simulink library "cooling_lib"  (R2022b)
settings: Solver=VariableStepAuto  StartTime=0.0  StopTime=10.0  RelTol=1e-3
undefined symbols (not defined in the file): raptor_get_param_eval, raptor_xcp_function
libraries: Raptor_lib x18, simulink x6
settings Model: Creator=serga  LastModifiedBy=serga

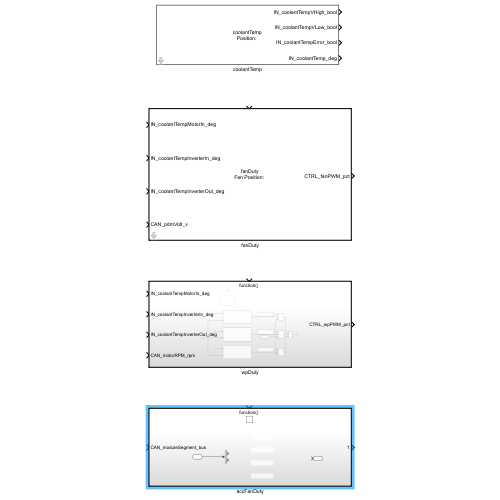
[thumbnail: Simulink's stored preview of the top-level diagram]
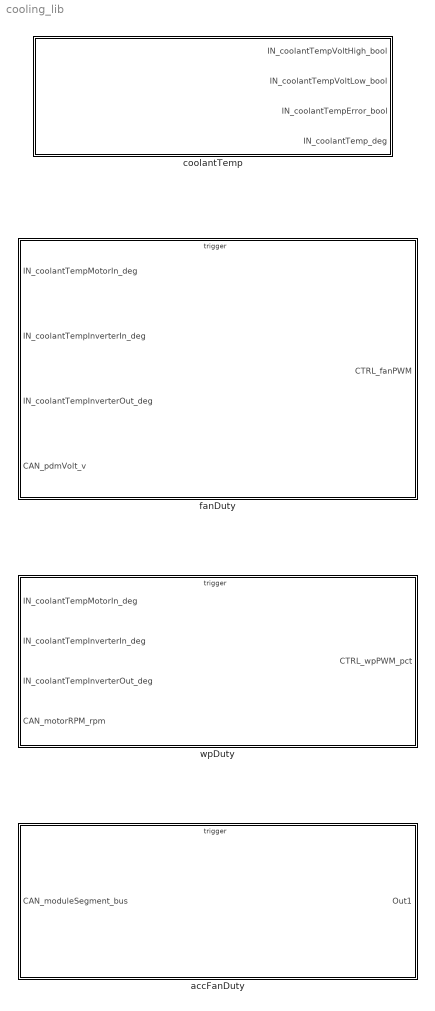
== system cooling_lib ==
  accFanDuty : Subsystem
  coolantTemp : Subsystem  mask{pos=''}
      mask prompts: pos "Position"
      mask Display:
      | disp(['coolantTemp\n'...
      |     'Position: ' pos]);
      | port_label('output', 1, ['IN_coolantTempVHigh' pos '_bool']);
      | port_label('output', 2, ['IN_coolantTempVLow' pos '_bool']);
      | port_label('output', 3, ['IN_coolantTempError' pos '_bool']);
      | port_label('output', 4, ['IN_coolantTemp' pos '_deg']);
  fanDuty : Subsystem  mask{pos=''}
      mask prompts: pos "Position"
      mask Display:
      | disp(['fanDuty\n'...
      |     'Fan Position: ' pos]);
      | port_label('input', 1, 'IN_coolantTempMotorIn_deg');
      | port_label('input', 2, 'IN_coolantTempInverterIn_deg');
      | port_label('input', 3, 'IN_coolantTempInverterOut_deg');
      | port_label('input', 4, 'CAN_pdmVolt_v');
      | port_label('output', 1, ['CTRL_fan' pos 'PWM_pct']);
  wpDuty : Subsystem

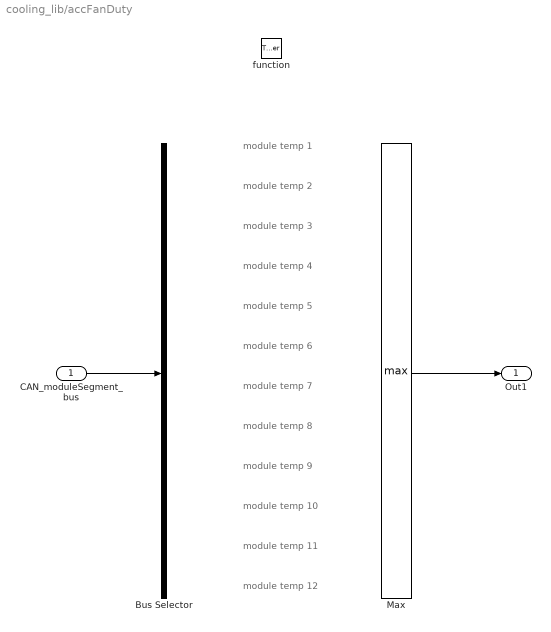
== system cooling_lib/accFanDuty ==
  note: module temp 1
  note: module temp 2
  note: module temp 3
  note: module temp 4
  note: module temp 5
  note: module temp 6
  note: module temp 7
  note: module temp 8
  note: module temp 9
  note: module temp 10
  note: module temp 11
  note: module temp 12
  CAN_moduleSegment_bus : Inport
  function : TriggerPort  TriggerType=function-call  VariantControl=(inherit)
  Bus Selector : BusSelector  OutputSignals=signal1,signal2
  Max : MinMax  Function=max  Inputs=12
  Out1 : Outport
  wires:
  CAN_moduleSegment_bus/1 -> Bus Selector/1
  Max/1 -> Out1/1

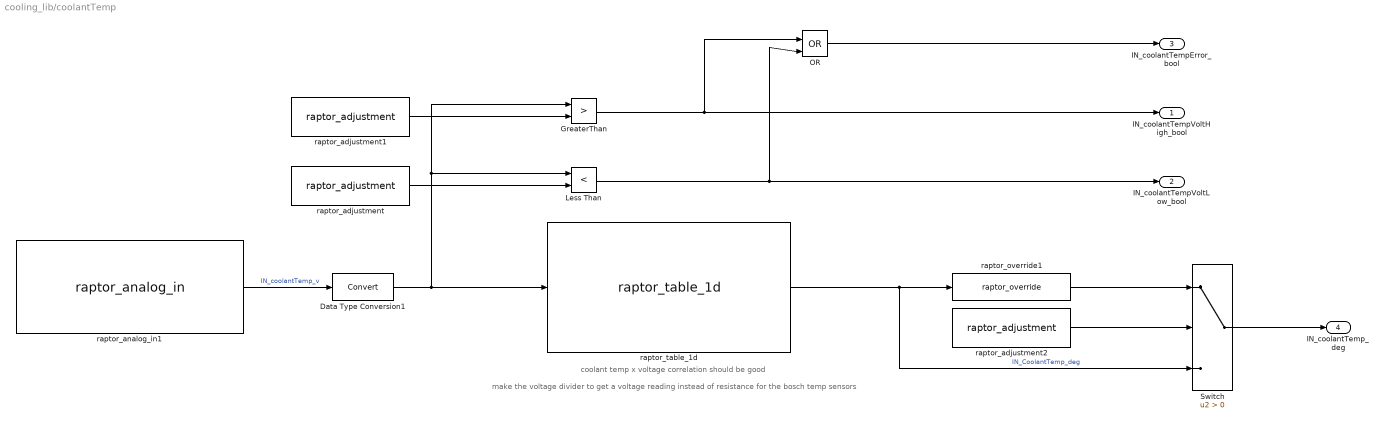
== system cooling_lib/coolantTemp ==
  note: coolant temp x voltage correlation should be good
  note: make the voltage divider to get a voltage reading instead of resistance for the bosch temp sensors
  Data Type Conversion1 : DataTypeConversion  SaturateOnIntegerOverflow=off  RndMeth=Floor
  GreaterThan : RelationalOperator  Operator=>  OutDataTypeStr=boolean  RndMeth=Simplest  InputSameDT=off
  Less Than : RelationalOperator  Operator=<  OutDataTypeStr=boolean  RndMeth=Simplest  InputSameDT=off
  OR : Logic  Operator=OR  IconShape=distinctive  AllPortsSameDT=off  OutDataTypeStr=boolean
  Switch : Switch  Criteria=u2 > Threshold  SaturateOnIntegerOverflow=off  InputSameDT=off
  raptor_adjustment : Raptor_lib/Data Storage/raptor_adjustment  paramName=['IN_coolantTempLow' pos '_v']  nameSource=Parameter  initValue=0.5  dataType=single  storage=Calibration  calDispType=Number  calEnum={'False', 'True'}  calGain=1.0  calOffset=0.0  calMax=inf  calMin=-inf  calFormat='-1'  calUnit=''  calHelp=''  calAccess=1  calFunction=raptor_xcp_function(gcb)  calDispHeaders=off  calColHeaders={'Col1' 'Col2' 'Col3'}  calRowHeaders={'Row1' 'Row2' 'Row3'}
      settings: SourceProductName=Raptor
  raptor_adjustment1 : Raptor_lib/Data Storage/raptor_adjustment  paramName=['IN_coolantTempHigh' pos '_v']  nameSource=Parameter  initValue=4.5  dataType=single  storage=Calibration  calDispType=Number  calEnum={'False', 'True'}  calGain=1.0  calOffset=0.0  calMax=inf  calMin=-inf  calFormat='-1'  calUnit=''  calHelp=''  calAccess=1  calFunction=raptor_xcp_function(gcb)  calDispHeaders=off  calColHeaders={'Col1' 'Col2' 'Col3'}  calRowHeaders={'Row1' 'Row2' 'Row3'}
      settings: SourceProductName=Raptor
  raptor_adjustment2 : Raptor_lib/Data Storage/raptor_adjustment  paramName=['IN_coolantTemp' pos '_bool']  nameSource=Parameter  initValue=0.00  dataType=boolean  storage=Calibration  calDispType=Number  calEnum={'False', 'True'}  calGain=1.0  calOffset=0.0  calMax=inf  calMin=-inf  calFormat='-1'  calUnit=''  calHelp=''  calAccess=1  calFunction=raptor_xcp_function(gcb)  calDispHeaders=off  calColHeaders={'Col1' 'Col2' 'Col3'}  calRowHeaders={'Row1' 'Row2' 'Row3'}
      settings: SourceProductName=Raptor
  raptor_analog_in1 : Raptor_lib/Input & Output/raptor_analog_in  resourceValues=INPUT2|INPUT3|INPUT4|INPUT5|INPUT6|INPUT7|INPUT8|INPUT9|INPUT10|INPUT11|INPUT12|INPUT13|INPUT14|INPUT15|INPUT16|INPUT17|INPUT18|INPUT19|INPUT20|INPUT21|INPUT22|INPUT23|INPUT24|INPUT25|INPUT26|INPUT27|INPUT28|INPUT29|INPUT30|INPUT31|INPUT32|(None)  resource=INPUT2  pullUDValues=2.15k PU  pullUD=2.15k PU  rangeValues=0 - 5 V  range=0 - 5 V  filterrateValues=[]  filterrate='RAPTOR MASK DEFAULT'  resolutionValues=[]  resolution=[]
      settings: SourceProductName=Raptor
  raptor_override1 : Raptor_lib/Data Storage/raptor_override  paramName=['IN_coolantTemp' pos '_deg']  nameSource=Parameter  measurement=Output  calDispType=Number  calEnum={'False', 'True'}  calGain=1.0  calOffset=0.0  calMax=inf  calMin=-inf  calFormat='-1'  calUnit=''  calHelp=''  calAccess=1  calFunction="[raptor_xcp_function(gcb) '|'  'Override']"
      settings: SourceProductName=Raptor
  raptor_table_1d : Raptor_lib/Table Lookup/raptor_table_1d  dataName=['IN_coolantTempVToDeg' pos]  initValue=[150 140 130 120 110 100 90 80 70 60 50 40 30 20 10 0 -10 -20 -30 -40]  dataType=double  storage=Calibration  initValueX=[0.2267 0.2793 0.3452 0.4303 0.5357 0.6741 0.8420 1.0604 1.3325 1.6592 2.0501 2.4737 2.9360 3.3784 3.7981 4.1545 4.4338 4.6399 4.7803 4.8710]  dataTypeXY=double  storageXY=Calibration  calVisible=on  showTable=on  calGain=1.0  calOffset=0.0  calMax=Inf  calMin=-Inf  calFormat='-1'  calUnit='Deg_C'  calHelp=''  showBreakpoint=on  dataNameX=[]  calGainX=1.0  calOffsetX=0.0  calMaxX=Inf  calMinX=-Inf  calFormatX='-1'  calUnitX='V'  calHelpX=''  calAccess=1  calFunction=raptor_xcp_function(gcb)  measureEnable=off  mName=['Data1D_Output']
      settings: SourceProductName=Raptor
  IN_coolantTempVoltHigh_bool : Outport  OutDataTypeStr=boolean
  IN_coolantTempVoltLow_bool : Outport  Port=2  OutDataTypeStr=boolean
  IN_coolantTempError_bool : Outport  Port=3  OutDataTypeStr=boolean
  IN_coolantTemp_deg : Outport  Port=4  OutDataTypeStr=double
  wires:
  raptor_override1/1 -> Switch/1
  OR/1 -> IN_coolantTempError_bool/1
  raptor_adjustment2/1 -> Switch/2
  raptor_analog_in1/1 -> Data Type Conversion1/1  "IN_coolantTemp_v"
  raptor_adjustment/1 -> Less Than/2
  raptor_table_1d/1 -> raptor_override1/1, Switch/3  "IN_CoolantTemp_deg"
  raptor_adjustment1/1 -> GreaterThan/2
  Switch/1 -> IN_coolantTemp_deg/1
  Less Than/1 -> IN_coolantTempVoltLow_bool/1, OR/2
  GreaterThan/1 -> OR/1, IN_coolantTempVoltHigh_bool/1
  Data Type Conversion1/1 -> GreaterThan/1, Less Than/1, raptor_table_1d/1

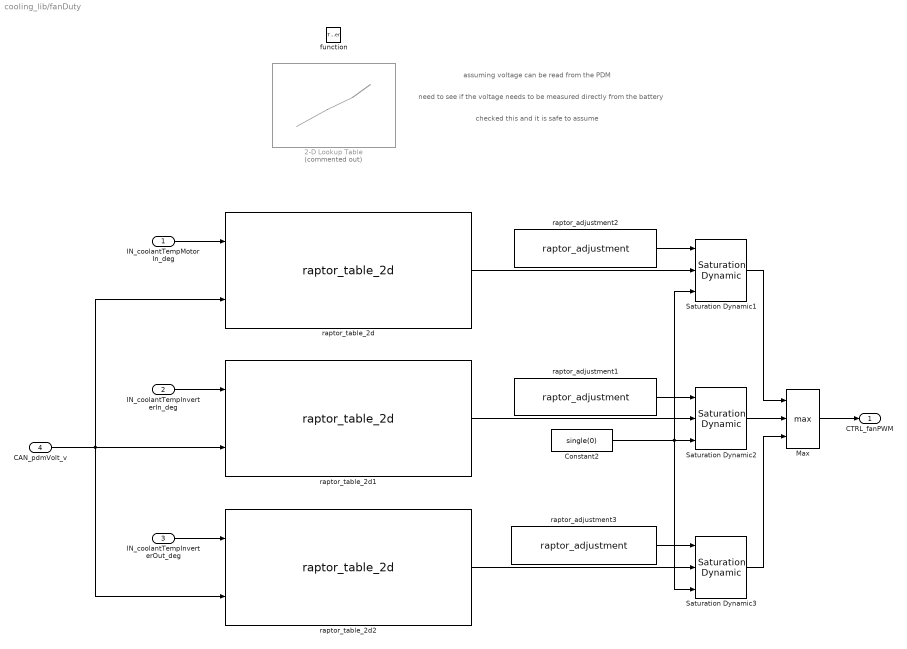
== system cooling_lib/fanDuty ==
  note: checked this and it is safe to assume
  note: need to see if the voltage needs to be measured directly from the battery
  note: assuming voltage can be read from the PDM
  IN_coolantTempMotorIn_deg : Inport
  IN_coolantTempInverterIn_deg : Inport  Port=2
  IN_coolantTempInverterOut_deg : Inport  Port=3
  CAN_pdmVolt_v : Inport  Port=4
  function : TriggerPort  TriggerType=function-call  VariantControl=(inherit)
  2-D Lookup Table : Lookup_n-D  Commented=on  LookupTableObject=''  BreakpointsForDimension1=[0;60;75;75.1;82;82.1;85;85.1;100;100.1;150]  BreakpointsForDimension2=[0 8 9 10 10.5 11 11.9 12 13 13.7 13.8 13.9 14.2 14.5]  BreakpointsForDimension1FirstPoint=10  BreakpointsForDimension2FirstPoint=10  BreakpointsForDimension1Spacing=12  BreakpointsForDimension2Spacing=12  IndexSearchMethod=Evenly spaced points  Table=[0 0 0 0 0 0 0 0 0 0 0 0 0 0;0 0 0 0 0 0 0 0 0 0 0 0 0 0;0 0 0 0 0 0 0 0 0 0 0 0 0 25;0 15 15 15 15 15 15 15 15 15 30 30 30 30;0 15 15 15 15 15 15 15 15 15 50 50 50 50;0 15 15 15 25 25 25 25 25 25 65 65 65 65;0 75 75 75 75 75 75 75 75 75 75 75 75 75;0 100 100 100 100 100 100 100 100 100 100 100 100 100;0 100 100 100 100 100 100 100 100 100 100 100 100 100;0 100 100 100 100 100 100 100 100 100 100 100 100 100;0 100 100 100 100 100 100 100 100 100 100 100 100 100]  InterpMethod=Flat  DiagnosticForOutOfRangeInput=Error  InternalRulePriority=Speed  RndMeth=Simplest
      settings: InputPortMap=u0,u1
  Constant2 : Constant  Value=single(0)
  Max : MinMax  Function=max  Inputs=3
  Saturation Dynamic1 : simulink/Discontinuities/Saturation Dynamic  OutMin=[]  OutMax=[]  OutDataTypeStr=Inherit: Same as second input  OutDataType=fixdt(1, 16)  OutScaling=2^-10  DoSatur=off
  Saturation Dynamic2 : simulink/Discontinuities/Saturation Dynamic  OutMin=[]  OutMax=[]  OutDataTypeStr=Inherit: Same as second input  OutDataType=fixdt(1, 16)  OutScaling=2^-10  DoSatur=off
  Saturation Dynamic3 : simulink/Discontinuities/Saturation Dynamic  OutMin=[]  OutMax=[]  OutDataTypeStr=Inherit: Same as second input  OutDataType=fixdt(1, 16)  OutScaling=2^-10  DoSatur=off
  raptor_adjustment1 : Raptor_lib/Data Storage/raptor_adjustment  paramName=['CTRL_upperThreshCoolantInverterIn' pos]  nameSource=Parameter  initValue=100  dataType=single  storage=Calibration  calDispType=Number  calEnum={'False', 'True'}  calGain=1.0  calOffset=0.0  calMax=inf  calMin=-inf  calFormat='-1'  calUnit=''  calHelp=''  calAccess=1  calFunction=raptor_xcp_function(gcb)  calDispHeaders=off  calColHeaders={'Col1' 'Col2' 'Col3'}  calRowHeaders={'Row1' 'Row2' 'Row3'}
      settings: SourceProductName=Raptor
  raptor_adjustment2 : Raptor_lib/Data Storage/raptor_adjustment  paramName=['CTRL_upperThreshCoolantMotorIn' pos]  nameSource=Parameter  initValue=100  dataType=single  storage=Calibration  calDispType=Number  calEnum={'False', 'True'}  calGain=1.0  calOffset=0.0  calMax=inf  calMin=-inf  calFormat='-1'  calUnit=''  calHelp=''  calAccess=1  calFunction=raptor_xcp_function(gcb)  calDispHeaders=off  calColHeaders={'Col1' 'Col2' 'Col3'}  calRowHeaders={'Row1' 'Row2' 'Row3'}
      settings: SourceProductName=Raptor
  raptor_adjustment3 : Raptor_lib/Data Storage/raptor_adjustment  paramName=['CTRL_upperThreshCoolantInverterOut' pos]  nameSource=Parameter  initValue=100  dataType=single  storage=Calibration  calDispType=Number  calEnum={'False', 'True'}  calGain=1.0  calOffset=0.0  calMax=inf  calMin=-inf  calFormat='-1'  calUnit=''  calHelp=''  calAccess=1  calFunction=raptor_xcp_function(gcb)  calDispHeaders=off  calColHeaders={'Col1' 'Col2' 'Col3'}  calRowHeaders={'Row1' 'Row2' 'Row3'}
      settings: SourceProductName=Raptor
  raptor_table_2d : Raptor_lib/Table Lookup/raptor_table_2d  dataName=['CTRL_coolantTempMotorInTo' pos 'Duty']  initValue=[0 0 0 0 0 0 0 0 0 0 0 0 0 0;0 0 0 0 0 0 0 0 0 0 0 0 0 0;0 0 0 0 0 0 0 0 0 0 0 0 0 25;0 15 15 15 15 15 15 15 15 15 30 30 30 30;0 15 15 15 15 15 15 15 15 15 50 50 50 50;0 15 15 15 25 25 25 25 25 25 65 65 65 65;0 75 75 75 75 75 75 75 75 75 75 75 75 75;0 100 100 100 100 100 100 100 100 100 100 100 100 100;0 100 100 100 100 100 100 100 100 100 100 100 100 100;0 100 100 100 100 100 100 100 100 100 100 100 100 100;0 100 100 100 100 100 100 100 100 100 100 100 100 100]  dataType=double  storage=Calibration  initValueX=[0 8 9 10 10.5 11 11.9 12 13 13.7 13.8 13.9 14.2 14.5]  initValueY=[0;60;75;75.1;82;82.1;85;85.1;100;100.1;150]  dataTypeXY=double  storageXY=Calibration  calVisible=on  showTable=off  calGain=1.0  calOffset=0.0  calMax=Inf  calMin=-Inf  calFormat='-1'  calUnit=''  calHelp=''  showBreakpointX=on  dataNameX=[]  calGainX=1.0  calOffsetX=0.0  calMaxX=Inf  calMinX=-Inf  calFormatX='-1'  calUnitX='pdmVolt'  calHelpX=''  showBreakpointY=on  dataNameY=[]  calGainY=1.0  calOffsetY=0.0  calMaxY=Inf  calMinY=-Inf  calFormatY='-1'  calUnitY='degC'  calHelpY=''  calAccess=1  calFunction=raptor_xcp_function(gcb)  measureEnable=off  mName=[raptor_get_param_eval(gcb,'dataName'), '_Output']
      settings: SourceProductName=Raptor
  raptor_table_2d1 : Raptor_lib/Table Lookup/raptor_table_2d  dataName=['CTRL_coolantTempInverterInTo' pos 'Duty']  initValue=[0 0 0 0 0 0 0 0 0 0 0 0 0 0;0 0 0 0 0 0 0 0 0 0 0 0 0 0;0 0 0 0 0 0 0 0 0 0 0 0 0 25;0 15 15 15 15 15 15 15 15 15 30 30 30 30;0 15 15 15 15 15 15 15 15 15 50 50 50 50;0 15 15 15 25 25 25 25 25 25 65 65 65 65;0 75 75 75 75 75 75 75 75 75 75 75 75 75;0 100 100 100 100 100 100 100 100 100 100 100 100 100;0 100 100 100 100 100 100 100 100 100 100 100 100 100;0 100 100 100 100 100 100 100 100 100 100 100 100 100;0 100 100 100 100 100 100 100 100 100 100 100 100 100]  dataType=double  storage=Calibration  initValueX=[0 8 9 10 10.5 11 11.9 12 13 13.7 13.8 13.9 14.2 14.5]  initValueY=[0;60;75;75.1;82;82.1;85;85.1;100;100.1;150]  dataTypeXY=double  storageXY=Calibration  calVisible=on  showTable=off  calGain=1.0  calOffset=0.0  calMax=Inf  calMin=-Inf  calFormat='-1'  calUnit=''  calHelp=''  showBreakpointX=on  dataNameX=[]  calGainX=1.0  calOffsetX=0.0  calMaxX=Inf  calMinX=-Inf  calFormatX='-1'  calUnitX='pdmVolt'  calHelpX=''  showBreakpointY=on  dataNameY=[]  calGainY=1.0  calOffsetY=0.0  calMaxY=Inf  calMinY=-Inf  calFormatY='-1'  calUnitY='degC'  calHelpY=''  calAccess=1  calFunction=raptor_xcp_function(gcb)  measureEnable=off  mName=[raptor_get_param_eval(gcb,'dataName'), '_Output']
      settings: SourceProductName=Raptor
  raptor_table_2d2 : Raptor_lib/Table Lookup/raptor_table_2d  dataName=['CTRL_coolantTempInverterOutTo' pos 'Duty']  initValue=[0 0 0 0 0 0 0 0 0 0 0 0 0 0;0 0 0 0 0 0 0 0 0 0 0 0 0 0;0 0 0 0 0 0 0 0 0 0 0 0 0 25;0 15 15 15 15 15 15 15 15 15 30 30 30 30;0 15 15 15 15 15 15 15 15 15 50 50 50 50;0 15 15 15 25 25 25 25 25 25 65 65 65 65;0 75 75 75 75 75 75 75 75 75 75 75 75 75;0 100 100 100 100 100 100 100 100 100 100 100 100 100;0 100 100 100 100 100 100 100 100 100 100 100 100 100;0 100 100 100 100 100 100 100 100 100 100 100 100 100;0 100 100 100 100 100 100 100 100 100 100 100 100 100]  dataType=double  storage=Calibration  initValueX=[0 8 9 10 10.5 11 11.9 12 13 13.7 13.8 13.9 14.2 14.5]  initValueY=[0;60;75;75.1;82;82.1;85;85.1;100;100.1;150]  dataTypeXY=double  storageXY=Calibration  calVisible=on  showTable=off  calGain=1.0  calOffset=0.0  calMax=Inf  calMin=-Inf  calFormat='-1'  calUnit=''  calHelp=''  showBreakpointX=on  dataNameX=[]  calGainX=1.0  calOffsetX=0.0  calMaxX=Inf  calMinX=-Inf  calFormatX='-1'  calUnitX='pdmVolt'  calHelpX=''  showBreakpointY=on  dataNameY=[]  calGainY=1.0  calOffsetY=0.0  calMaxY=Inf  calMinY=-Inf  calFormatY='-1'  calUnitY='degC'  calHelpY=''  calAccess=1  calFunction=raptor_xcp_function(gcb)  measureEnable=off  mName=[raptor_get_param_eval(gcb,'dataName'), '_Output']
      settings: SourceProductName=Raptor
  CTRL_fanPWM : Outport
  wires:
  IN_coolantTempMotorIn_deg/1 -> raptor_table_2d/1
  IN_coolantTempInverterIn_deg/1 -> raptor_table_2d1/1
  IN_coolantTempInverterOut_deg/1 -> raptor_table_2d2/1
  CAN_pdmVolt_v/1 -> raptor_table_2d/2, raptor_table_2d1/2, raptor_table_2d2/2
  Max/1 -> CTRL_fanPWM/1
  raptor_table_2d/1 -> Saturation Dynamic1/2
  Saturation Dynamic1/1 -> Max/1
  Saturation Dynamic2/1 -> Max/2
  raptor_table_2d1/1 -> Saturation Dynamic2/2
  raptor_table_2d2/1 -> Saturation Dynamic3/2
  Saturation Dynamic3/1 -> Max/3
  Constant2/1 -> Saturation Dynamic1/3, Saturation Dynamic3/3, Saturation Dynamic2/3
  raptor_adjustment2/1 -> Saturation Dynamic1/1
  raptor_adjustment1/1 -> Saturation Dynamic2/1
  raptor_adjustment3/1 -> Saturation Dynamic3/1

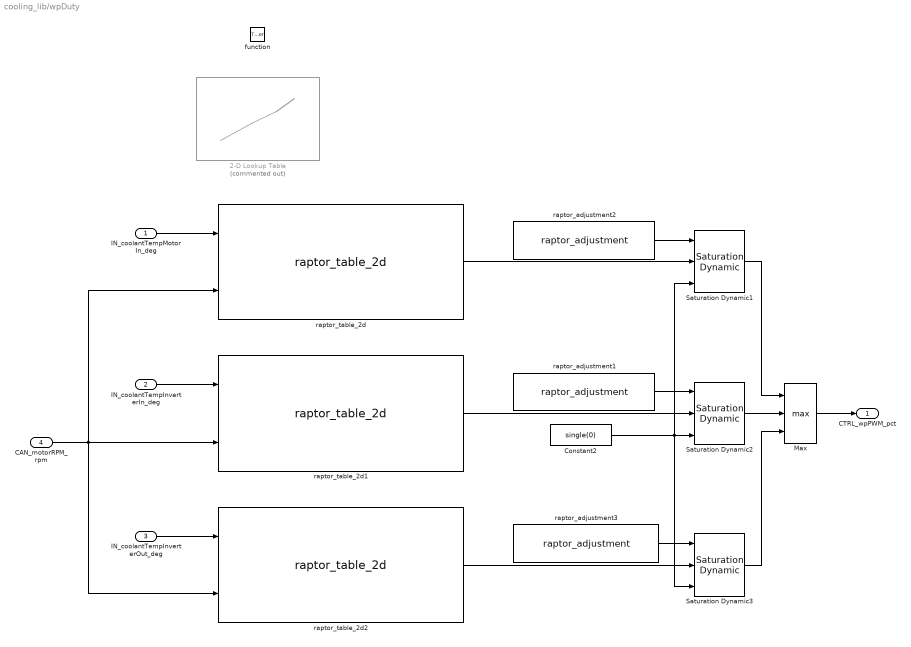
== system cooling_lib/wpDuty ==
  IN_coolantTempMotorIn_deg : Inport
  IN_coolantTempInverterIn_deg : Inport  Port=2
  IN_coolantTempInverterOut_deg : Inport  Port=3
  CAN_motorRPM_rpm : Inport  Port=4
  function : TriggerPort  TriggerType=function-call  VariantControl=(inherit)
  2-D Lookup Table : Lookup_n-D  Commented=on  LookupTableObject=''  BreakpointsForDimension1=[10;20;40;50;60;69.9;70;84.5;84.6;100;150]  BreakpointsForDimension2=[0;0;10;20;500;510;5000;15000]  BreakpointsForDimension1FirstPoint=10  BreakpointsForDimension2FirstPoint=10  BreakpointsForDimension1Spacing=12  BreakpointsForDimension2Spacing=12  IndexSearchMethod=Evenly spaced points  Table=[0 0 0 0 0 20 20 0;0 0 0 0 0 20 20 0;0 0 0 0 0 35 35 15;0 0 0 0 0 35 35 15;0 0 0 0 0 35 35 25;0 0 0 0 0 35 35 75;0 0 0 0 0 40 40 40;0 0 0 0 0 50 50 50;0 0 25 0 0 60 60 60;0 0 100 0 0 100 100 100;0 0 100 0 0 100 100 100]  InterpMethod=Flat  DiagnosticForOutOfRangeInput=Error  InternalRulePriority=Speed  RndMeth=Simplest
      settings: InputPortMap=u0,u1
  Constant2 : Constant  Value=single(0)
  Max : MinMax  Function=max  Inputs=3
  Saturation Dynamic1 : simulink/Discontinuities/Saturation Dynamic  OutMin=[]  OutMax=[]  OutDataTypeStr=Inherit: Same as second input  OutDataType=fixdt(1, 16)  OutScaling=2^-10  DoSatur=off
  Saturation Dynamic2 : simulink/Discontinuities/Saturation Dynamic  OutMin=[]  OutMax=[]  OutDataTypeStr=Inherit: Same as second input  OutDataType=fixdt(1, 16)  OutScaling=2^-10  DoSatur=off
  Saturation Dynamic3 : simulink/Discontinuities/Saturation Dynamic  OutMin=[]  OutMax=[]  OutDataTypeStr=Inherit: Same as second input  OutDataType=fixdt(1, 16)  OutScaling=2^-10  DoSatur=off
  raptor_adjustment1 : Raptor_lib/Data Storage/raptor_adjustment  paramName='CTRL_upperThreshCoolantInverterIn'  nameSource=Parameter  initValue=100  dataType=single  storage=Calibration  calDispType=Number  calEnum={'False', 'True'}  calGain=1.0  calOffset=0.0  calMax=inf  calMin=-inf  calFormat='-1'  calUnit=''  calHelp=''  calAccess=1  calFunction=raptor_xcp_function(gcb)  calDispHeaders=off  calColHeaders={'Col1' 'Col2' 'Col3'}  calRowHeaders={'Row1' 'Row2' 'Row3'}
      settings: SourceProductName=Raptor
  raptor_adjustment2 : Raptor_lib/Data Storage/raptor_adjustment  paramName='CTRL_upperThreshCoolantMotorIn'  nameSource=Parameter  initValue=100  dataType=single  storage=Calibration  calDispType=Number  calEnum={'False', 'True'}  calGain=1.0  calOffset=0.0  calMax=inf  calMin=-inf  calFormat='-1'  calUnit=''  calHelp=''  calAccess=1  calFunction=raptor_xcp_function(gcb)  calDispHeaders=off  calColHeaders={'Col1' 'Col2' 'Col3'}  calRowHeaders={'Row1' 'Row2' 'Row3'}
      settings: SourceProductName=Raptor
  raptor_adjustment3 : Raptor_lib/Data Storage/raptor_adjustment  paramName='CTRL_upperThreshCoolantInverterOut'  nameSource=Parameter  initValue=100  dataType=single  storage=Calibration  calDispType=Number  calEnum={'False', 'True'}  calGain=1.0  calOffset=0.0  calMax=inf  calMin=-inf  calFormat='-1'  calUnit=''  calHelp=''  calAccess=1  calFunction=raptor_xcp_function(gcb)  calDispHeaders=off  calColHeaders={'Col1' 'Col2' 'Col3'}  calRowHeaders={'Row1' 'Row2' 'Row3'}
      settings: SourceProductName=Raptor
  raptor_table_2d : Raptor_lib/Table Lookup/raptor_table_2d  dataName='CTRL_coolantTempMotorInToWpDuty'  initValue=[0 0 0 0 0 20 20 0;0 0 0 0 0 20 20 0;0 0 0 0 0 35 35 15;0 0 0 0 0 35 35 15;0 0 0 0 0 35 35 25;0 0 0 0 0 35 35 75;0 0 0 0 0 40 40 40;0 0 0 0 0 50 50 50;0 0 25 0 0 60 60 60;0 0 100 0 0 100 100 100;0 0 100 0 0 100 100 100]  dataType=double  storage=Calibration  initValueX=[0;0;10;20;500;510;5000;15000]  initValueY=[10;20;40;50;60;69.9;70;84.5;84.6;100;150]  dataTypeXY=double  storageXY=Calibration  calVisible=on  showTable=off  calGain=1.0  calOffset=0.0  calMax=Inf  calMin=-Inf  calFormat='-1'  calUnit=''  calHelp=''  showBreakpointX=on  dataNameX=[]  calGainX=1.0  calOffsetX=0.0  calMaxX=Inf  calMinX=-Inf  calFormatX='-1'  calUnitX='motorRPM'  calHelpX=''  showBreakpointY=on  dataNameY=[]  calGainY=1.0  calOffsetY=0.0  calMaxY=Inf  calMinY=-Inf  calFormatY='-1'  calUnitY='degC'  calHelpY=''  calAccess=1  calFunction=raptor_xcp_function(gcb)  measureEnable=off  mName=[raptor_get_param_eval(gcb,'dataName'), '_Output']
      settings: SourceProductName=Raptor
  raptor_table_2d1 : Raptor_lib/Table Lookup/raptor_table_2d  dataName='CTRL_coolantTempInverterInToWpDuty'  initValue=[0 0 0 0 0 20 20 0;0 0 0 0 0 20 20 0;0 0 0 0 0 35 35 15;0 0 0 0 0 35 35 15;0 0 0 0 0 35 35 25;0 0 0 0 0 35 35 75;0 0 0 0 0 40 40 40;0 0 0 0 0 50 50 50;0 0 25 0 0 60 60 60;0 0 100 0 0 100 100 100;0 0 100 0 0 100 100 100]  dataType=double  storage=Calibration  initValueX=[0;0;10;20;500;510;5000;15000]  initValueY=[10;20;40;50;60;69.9;70;84.5;84.6;100;150]  dataTypeXY=double  storageXY=Calibration  calVisible=on  showTable=off  calGain=1.0  calOffset=0.0  calMax=Inf  calMin=-Inf  calFormat='-1'  calUnit=''  calHelp=''  showBreakpointX=on  dataNameX=[]  calGainX=1.0  calOffsetX=0.0  calMaxX=Inf  calMinX=-Inf  calFormatX='-1'  calUnitX='motorRPM'  calHelpX=''  showBreakpointY=on  dataNameY=[]  calGainY=1.0  calOffsetY=0.0  calMaxY=Inf  calMinY=-Inf  calFormatY='-1'  calUnitY='degC'  calHelpY=''  calAccess=1  calFunction=raptor_xcp_function(gcb)  measureEnable=off  mName=[raptor_get_param_eval(gcb,'dataName'), '_Output']
      settings: SourceProductName=Raptor
  raptor_table_2d2 : Raptor_lib/Table Lookup/raptor_table_2d  dataName='CTRL_coolantTempInverterOutToWpDuty'  initValue=[0 0 0 0 0 20 20 0;0 0 0 0 0 20 20 0;0 0 0 0 0 35 35 15;0 0 0 0 0 35 35 15;0 0 0 0 0 35 35 25;0 0 0 0 0 35 35 75;0 0 0 0 0 40 40 40;0 0 0 0 0 50 50 50;0 0 25 0 0 60 60 60;0 0 100 0 0 100 100 100;0 0 100 0 0 100 100 100]  dataType=double  storage=Calibration  initValueX=[0;0;10;20;500;510;5000;15000]  initValueY=[10;20;40;50;60;69.9;70;84.5;84.6;100;150]  dataTypeXY=double  storageXY=Calibration  calVisible=on  showTable=off  calGain=1.0  calOffset=0.0  calMax=Inf  calMin=-Inf  calFormat='-1'  calUnit=''  calHelp=''  showBreakpointX=on  dataNameX=[]  calGainX=1.0  calOffsetX=0.0  calMaxX=Inf  calMinX=-Inf  calFormatX='-1'  calUnitX='motorRPM'  calHelpX=''  showBreakpointY=on  dataNameY=[]  calGainY=1.0  calOffsetY=0.0  calMaxY=Inf  calMinY=-Inf  calFormatY='-1'  calUnitY='degC'  calHelpY=''  calAccess=1  calFunction=raptor_xcp_function(gcb)  measureEnable=off  mName=[raptor_get_param_eval(gcb,'dataName'), '_Output']
      settings: SourceProductName=Raptor
  CTRL_wpPWM_pct : Outport
  wires:
  IN_coolantTempMotorIn_deg/1 -> raptor_table_2d/1
  IN_coolantTempInverterIn_deg/1 -> raptor_table_2d1/1
  IN_coolantTempInverterOut_deg/1 -> raptor_table_2d2/1
  CAN_motorRPM_rpm/1 -> raptor_table_2d2/2, raptor_table_2d1/2, raptor_table_2d/2
  raptor_adjustment1/1 -> Saturation Dynamic2/1
  Saturation Dynamic2/1 -> Max/2
  Saturation Dynamic1/1 -> Max/1
  Max/1 -> CTRL_wpPWM_pct/1
  raptor_table_2d1/1 -> Saturation Dynamic2/2
  raptor_adjustment2/1 -> Saturation Dynamic1/1
  raptor_table_2d2/1 -> Saturation Dynamic3/2
  Constant2/1 -> Saturation Dynamic2/3, Saturation Dynamic1/3, Saturation Dynamic3/3
  raptor_table_2d/1 -> Saturation Dynamic1/2
  Saturation Dynamic3/1 -> Max/3
  raptor_adjustment3/1 -> Saturation Dynamic3/1
